simulink model "am"  (R2018b)
settings: Solver=VariableStepAuto  StartTime=0.0  StopTime=20  RelTol=1e-3
libraries: commanapbnd3 x1
settings Model: Creator=trevor  LastModifiedBy=trevor

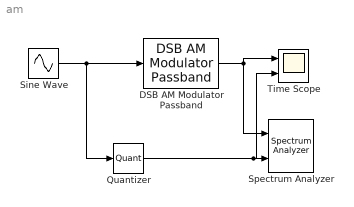
== system am ==
  DSB AM Modulator Passband : commanapbnd3/DSB AM Modulator Passband  Fc=20  Ph=0  Offset=0
      settings: SourceProductName=Communications System Toolbox  SourceProductBaseCode=CM
  Quantizer : Quantizer  QuantizationInterval=0.05
  Sine Wave : Sin  SineType=Sample based  Samples=100  SampleTime=0.01
  Spectrum Analyzer : SpectrumAnalyzer  NumInputPorts=2
  Time Scope : Scope  NumInputPorts=2
  wires:
  Sine Wave/1 -> Quantizer/1, DSB AM Modulator Passband/1
  DSB AM Modulator Passband/1 -> Spectrum Analyzer/1, Time Scope/1
  Quantizer/1 -> Time Scope/2, Spectrum Analyzer/2
